simulink library "speedgoatlib_fpga_analog_io"  (R2024b)
settings: Solver=VariableStepAuto  StartTime=0.0  StopTime=10.0  RelTol=1e-3
undefined symbols (not defined in the file): IO336, sg_fpga_callBackInit_m_a1, sg_fpga_io324_analog_input_m, sg_fpga_io324_analog_output_m, sg_fpga_io324_analog_setup_m, sg_fpga_io325_analog_input_m, sg_fpga_io325_analog_output_m, sg_fpga_io325_analog_setup_m, sg_fpga_io334_analog_input_m, sg_fpga_io334_analog_output_m, sg_fpga_io334_analog_setup_m, sg_fpga_io336_analog_input_m, sg_fpga_io336_analog_output_m, sg_fpga_io336_analog_setup_m, sg_fpga_io337_analog_input_m, sg_fpga_io337_analog_output_m, sg_fpga_io337_analog_setup_m, sg_fpga_io3xx_120_analog_input_m, sg_fpga_io3xx_120_analog_output_m, sg_fpga_io3xx_120_analog_setup_m
(part 2 of 4)

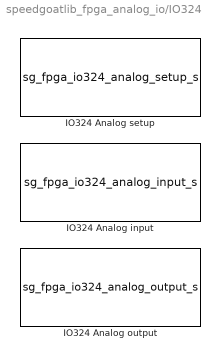
== system speedgoatlib_fpga_analog_io/IO324 ==
  IO324 Analog input : S-Function  InitFcn=sg_fpga_io324_analog_input_m.runInitFcn();  FunctionName=sg_fpga_io324_analog_input_s  Parameters=id, parSampleTime, parAiChannels, parAiVoltageRange, parAiTriggerMode, parAiReadPrevValue, parAiEnableFrame, parAiFrameSize  SFunctionDeploymentMode=off  EnableBusSupport=off  mask(ad_fpga_IO324){id=1, parSampleTime=-1, parPciSlot=-1, parAiChannels=[1 2], parAiTriggerMode=[2 2 2 2], parAiReadPrevValue=0, parAiEnableFrame=0, parAiVoltageRange=[3 3], parAdcCoupling=[1 1 1 1], parAdcContSampling=0, parAdcDmaEnable=0, parAdcActiveDmaDevices=[1 1 1 1], parAiFrameSize=100}
      mask prompts: id "Configurable I/O Module ID"; parSampleTime "Sample Time [s]"
      mask help: Speedgoat Driver Block<br>IO324-200k - IO324 Analog Input<br><br>&copy; 2007 - 2026, Speedgoat GmbH, <a href="matlab: web('www.speedgoat.com','-browser');">www.speedgoat.com</a>
      mask init:
      | sg_fpga_io324_analog_input_m.runMaskInit();
      mask Help: eval('sg.utils.help.show(''io_main/refentry_io324_analog_input_v1'');')
      mask TypeOptions id: 1 | 2 | 3 | 4 | 5 | 6 | 7 | 8 | 9 | 10
      mask Display: disp('Speedgoat\nIO324-200k\nAnalog input v1\nModule ID: 1');port_label('output',1,'1');port_label('output',2,'2');
  IO324 Analog output : S-Function  InitFcn=sg_fpga_io324_analog_output_m.runInitFcn();  FunctionName=sg_fpga_io324_analog_output_s  Parameters=id, parSampleTime, parAoChannels, parAoVoltageRange, parAoInitValues, parAoReset, parAoEnableFrame, parAoFrameSize  SFunctionDeploymentMode=off  EnableBusSupport=off  mask(da_fpga_IO324){id=1, parSampleTime=-1, parPciSlot=-1, parAoChannels=[1 2], parAoVoltageRange=[2 2], parDacOverRange=[0 0 0 0 0 0 0 0], parAoInitValues=[0 0], parAoReset=[1 1], parDacSyncOut=1, parAoEnableFrame=0, parDacActiveDmaDevices=[1 1 1 1], parDacDmaLatency=2, parAoFrameSize=1000}
      mask prompts: id "Configurable I/O Module ID"; parSampleTime "Sample Time [s]"
      mask help: Speedgoat Driver Block<br>IO324-200k - IO324 Analog Output<br><br>&copy; 2007 - 2026, Speedgoat GmbH, <a href="matlab: web('www.speedgoat.com','-browser');">www.speedgoat.com</a>
      mask init:
      | sg_fpga_io324_analog_output_m.runMaskInit();
      mask Help: eval('sg.utils.help.show(''io_main/refentry_io324_analog_output_v1'');')
      mask TypeOptions id: 1 | 2 | 3 | 4 | 5 | 6 | 7 | 8 | 9 | 10
      mask Display: disp('Speedgoat\nIO324-200k\nAnalog output v1\nModule ID: 1');port_label('input',1,'1');port_label('input',2,'2');
  IO324 Analog setup : S-Function  InitFcn=sg_fpga_io324_analog_setup_m.runInitFcn();  FunctionName=sg_fpga_io324_analog_setup_s  Parameters=id, p.AdcActiveChannels, p.AdcCoupling, p.AdcVoltageRange, p.AdcFilterWidthPow2, p.AdcOversamplRate, parAdcAutoCorrection, p.AdcTriggerMode, p.AdcClockDivider, p.AdcInternalTrigger, p.AdcExternalTrigger, p.AdcEnableFrame, p.AdcFrameSize, p.DacChannels, p.DacVoltageRange, p.DacInitValues, p.DacReset, parDacAutoCorrection, p.DacTriggerMode, p.DacClockDivider, p.DacInternalTrigger, p.DacExternalTrigger, p.DacEnableFrame, p.DacFifoThreshold, p.DacSourceSelection, p.EnableTriggerForCm,p.DacUsesTimer  SFunctionModules=sg_fpga_analog_dma sg_AnalogInputCm_IO324 sg_AnalogOutputCm  SFunctionDeploymentMode=off  EnableBusSupport=off  mask(analog_setup_fpga_IO324){id=1, parEnableCodeModule1=off, parEnableCodeModule2=off, parEnableCodeModule3=off, parEnableCodeModule4=off, parEnableCodeModule5=off, parEnableCodeModule6=off, parEnableCodeModule7=off, parEnableCodeModule8=off, parAdcEnableIndividualTrigger=off, parAdcTriggerMode1=Model Step, parAdcSampleRate1=100e3, parAdcDioTriggerChannel1=1, parAdcInternalTrigger1=<empty>, parAdcOversampling1=None, parAdcTriggerMode2=Model Step, parAdcSampleRate2=100e3, parAdcDioTriggerChannel2=1, parAdcInternalTrigger2=<empty>, parAdcOversampling2=None, parAdcTriggerMode3=Model Step, parAdcSampleRate3=100e3, parAdcDioTriggerChannel3=1, parAdcInternalTrigger3=<empty>, parAdcOversampling3=None, parAdcTriggerMode4=Model Step, parAdcSampleRate4=100e3, parAdcDioTriggerChannel4=1, parAdcInternalTrigger4=<empty>, parAdcOversampling4=None, parAdcReadPrevValueIndividualTrigger=on, parAdcEnableFrame=off, parAdcTriggerMode=I/O Module Clock, parAdcReadPrevValue=on, parAdcSampleRate=100e3, parAdcDioTriggerChannel=1, parAdcInternalTrigger=<empty>, parAdcOversampling=None, parAdcTriggerResolution=1e-08, parAdcSampleRateFrame=100e3, parAdcFrameSize=100, parAdcSampleTime=-1, parDacTriggerMode=Model Step, parDacInternalTrigger=<empty>, parDacDioTriggerChannel=0, parDacEnableFrame=on, dacUsesTimer=off, parDacFifoThreshold=100, parDacTriggerResolution=1e-08, parDacSampleRate=1e6, parDacFrameSize=1000, parDacSampleTime=-1, parAdcCoupling1=Single-Ended, parAdcChannel1=on, parAdcChannel2=on, parAdcChannel3=off, parAdcChannel4=off, parAdcChannel5=off, parAdcChannel6=off, parAdcChannel7=off, parAdcChannel8=off, parAdcRangeAll1=+-5.12 V, parVoltageRangePerChannelEn1=off, parAdcRange1=+-5.12 V, parAdcRange5=+-5.12 V, parAdcRange2=+-5.12 V, parAdcRange6=+-5.12 V, parAdcRange3=+-5.12 V, parAdcRange7=+-5.12 V, parAdcRange4=+-5.12 V, parAdcRange8=+-5.12 V, parAdcCoupling2=Single-Ended, parAdcChannel9=off, parAdcChannel10=off, parAdcChannel11=off, parAdcChannel12=off, parAdcChannel13=off, parAdcChannel14=off, parAdcChannel15=off, parAdcChannel16=off, parAdcRangeAll2=+-5.12 V, parVoltageRangePerChannelEn2=off, parAdcRange9=+-5.12 V, parAdcRange13=+-5.12 V, parAdcRange10=+-5.12 V, parAdcRange14=+-5.12 V, parAdcRange11=+-5.12 V, parAdcRange15=+-5.12 V, parAdcRange12=+-5.12 V, parAdcRange16=+-5.12 V, parAdcCoupling3=Single-Ended, parAdcChannel17=off, parAdcChannel18=off, parAdcChannel19=off, parAdcChannel20=off, parAdcChannel21=off, parAdcChannel22=off, parAdcChannel23=off, parAdcChannel24=off, parAdcRangeAll3=+-5.12 V, parVoltageRangePerChannelEn3=off, parAdcRange17=+-5.12 V, parAdcRange21=+-5.12 V, parAdcRange18=+-5.12 V, parAdcRange22=+-5.12 V, parAdcRange19=+-5.12 V, parAdcRange23=+-5.12 V, parAdcRange20=+-5.12 V, parAdcRange24=+-5.12 V, parAdcCoupling4=Single-Ended, parAdcChannel25=off, parAdcChannel26=off, parAdcChannel27=off, parAdcChannel28=off, parAdcChannel29=off, parAdcChannel30=off, parAdcChannel31=off, parAdcChannel32=off, parAdcRangeAll4=+-5.12 V, parVoltageRangePerChannelEn4=off, parAdcRange25=+-5.12 V, parAdcRange29=+-5.12 V, parAdcRange26=+-5.12 V, parAdcRange30=+-5.12 V, parAdcRange27=+-5.12 V, parAdcRange31=+-5.12 V, parAdcRange28=+-5.12 V, parAdcRange32=+-5.12 V, parAdcAutoCorrection=on, parDacChannel1=on, parDacChannel2=on, parDacChannel3=off, parDacChannel4=off, parDacChannel5=off, parDacChannel6=off, parDacChannel7=off, parDacChannel8=off, parDacRange1=+-5 V, parDacInitValue1=0, parDacReset1=on, parDacRange2=+-5 V, parDacInitValue2=0, parDacReset2=on, parDacRange3=+-5 V, parDacInitValue3=0, parDacReset3=on, parDacRange4=+-5 V, parDacInitValue4=0, parDacReset4=on, parDacRange5=+-5 V, parDacInitValue5=0, parDacReset5=on, parDacRange6=+-5 V, parDacInitValue6=0, parDacReset6=on, parDacRange7=+-5 V, parDacInitValue7=0, parDacReset7=on, parDacRange8=+-5 V, parDacInitValue8=0, parDacReset8=on, parDacAutoCorrection=on}
      mask prompts: id "Configurable I/O Module ID"; parAdcEnableIndividualTrigger "Enable Individual Trigger Settings"; parAdcTriggerMode1 "ADC Sample Trigger"; parAdcSampleRate1 "ADC Sample Rate [Hz]"; parAdcDioTriggerChannel1 "Digital I/O Channel"; parAdcInternalTrigger1 "Internal Signal"; parAdcOversampling1 "Oversampling Factor"; parAdcTriggerMode2 "ADC Sample Trigger"; parAdcSampleRate2 "ADC Sample Rate [Hz]"; parAdcDioTriggerChannel2 "Digital I/O Channel"; parAdcInternalTrigger2 "Internal Signal"; parAdcOversampling2 "Oversampling Factor"; parAdcTriggerMode3 "ADC Sample Trigger"; parAdcSampleRate3 "ADC Sample Rate [Hz]"; parAdcDioTriggerChannel3 "Digital I/O Channel"; parAdcInternalTrigger3 "Internal Signal"; parAdcOversampling3 "Oversampling Factor"; parAdcTriggerMode4 "ADC Sample Trigger"; parAdcSampleRate4 "ADC Sample Rate [Hz]"; parAdcDioTriggerChannel4 "Digital I/O Channel"; parAdcInternalTrigger4 "Internal Signal"; parAdcOversampling4 "Oversampling Factor"; parAdcReadPrevValueIndividualTrigger "Read Value From Previous Model Step"; parAdcEnableFrame "Enable DMA Interrupt"; parAdcTriggerMode "ADC Sample Trigger"; parAdcReadPrevValue "Read Value From Previous Model Step"; parAdcSampleRate "ADC Sample Rate [Hz]"; parAdcDioTriggerChannel "Digital I/O Channel"; parAdcInternalTrigger "Internal Signal"; parAdcOversampling "Oversampling Factor"; parAdcTriggerResolution "Trigger Resolution [s]"; parAdcSampleRateFrame "ADC Sample Rate [Hz]"; parAdcFrameSize "Frame Size (samples/channel)"; parAdcSampleTime "Input Block Sample Time [s]"; parDacTriggerMode "DAC Sample Trigger"; parDacInternalTrigger "Internal Signal"; parDacDioTriggerChannel "Digital I/O Channel"; parDacEnableFrame "Enable DMA Interrupt"; dacUsesTimer "Set Sampling Frequency"; parDacFifoThreshold "FIFO Threshold (samples/channel)"; parDacTriggerResolution "Trigger Resolution [s]"; parDacSampleRate "DAC Sample Rate [Hz]"; parDacFrameSize "Frame Size (samples/channel)"; parDacSampleTime "Output Block Sample Time [s]"; parAdcCoupling1 "Signal Mode"; parAdcChannel1 "Ch 01"; parAdcChannel2 "Ch 02"; parAdcChannel3 "Ch 03"; parAdcChannel4 "Ch 04"; parAdcChannel5 "Ch 05"; parAdcChannel6 "Ch 06"; parAdcChannel7 "Ch 07"; parAdcChannel8 "Ch 08"; parAdcRangeAll1 "Voltage Range"; parVoltageRangePerChannelEn1 "Set Voltage Range per Channel"; parAdcRange1 "Ch 01"; parAdcRange5 "Ch 05"; parAdcRange2 "Ch 02"; parAdcRange6 "Ch 06"; parAdcRange3 "Ch 03"; parAdcRange7 "Ch 07"; parAdcRange4 "Ch 04"; parAdcRange8 "Ch 08"; parAdcCoupling2 "Signal Mode"; parAdcChannel9 "Ch 09"; parAdcChannel10 "Ch 10"; parAdcChannel11 "Ch 11"; parAdcChannel12 "Ch 12"; parAdcChannel13 "Ch 13"; parAdcChannel14 "Ch 14"; parAdcChannel15 "Ch 15"; parAdcChannel16 "Ch 16"; parAdcRangeAll2 "Voltage Range"; parVoltageRangePerChannelEn2 "Set Voltage Range per Channel"; parAdcRange9 "Ch 09"; parAdcRange13 "Ch 13"; parAdcRange10 "Ch 10"; parAdcRange14 "Ch 14"; parAdcRange11 "Ch 11"; parAdcRange15 "Ch 15"; parAdcRange12 "Ch 12"; parAdcRange16 "Ch 16"; parAdcCoupling3 "Signal Mode"; parAdcChannel17 "Ch 17"; parAdcChannel18 "Ch 18"; parAdcChannel19 "Ch 19"; parAdcChannel20 "Ch 20"; parAdcChannel21 "Ch 21"; parAdcChannel22 "Ch 22"; parAdcChannel23 "Ch 23"; parAdcChannel24 "Ch 24"; parAdcRangeAll3 "Voltage Range"; parVoltageRangePerChannelEn3 "Set Voltage Range per Channel"; parAdcRange17 "Ch 17"; parAdcRange21 "Ch 21"; parAdcRange18 "Ch 18"; parAdcRange22 "Ch 22"; parAdcRange19 "Ch 19"; parAdcRange23 "Ch 23"; parAdcRange20 "Ch 20"; parAdcRange24 "Ch 24"; parAdcCoupling4 "Signal Mode"; parAdcChannel25 "Ch 25"; parAdcChannel26 "Ch 26"; parAdcChannel27 "Ch 27"; parAdcChannel28 "Ch 28"; parAdcChannel29 "Ch 29"; parAdcChannel30 "Ch 30"; parAdcChannel31 "Ch 31"; parAdcChannel32 "Ch 32"; parAdcRangeAll4 "Voltage Range"; parVoltageRangePerChannelEn4 "Set Voltage Range per Channel"; parAdcRange25 "Ch 25"; parAdcRange29 "Ch 29"; parAdcRange26 "Ch 26"; parAdcRange30 "Ch 30"; parAdcRange27 "Ch 27"; parAdcRange31 "Ch 31"; parAdcRange28 "Ch 28"; parAdcRange32 "Ch 32"; parAdcAutoCorrection "Automatic Data Correction (for Debugging)"; parDacChannel1 "Ch 1"; parDacChannel2 "Ch 2"; parDacChannel3 "Ch 3"; parDacChannel4 "Ch 4"; parDacChannel5 "Ch 5"; parDacChannel6 "Ch 6"; parDacChannel7 "Ch 7"; parDacChannel8 "Ch 8"; parDacRange1 "Output Range"; parDacInitValue1 "Initial Value [V]"; parDacReset1 "Reset to Initial Value"; parDacRange2 "Output Range"; parDacInitValue2 "Initial Value [V]"; parDacReset2 "Reset to Initial Value"; parDacRange3 "Output Range"; parDacInitValue3 "Initial Value [V]"; parDacReset3 "Reset to Initial Value"; parDacRange4 "Output Range"; parDacInitValue4 "Initial Value [V]"; parDacReset4 "Reset to Initial Value"; parDacRange5 "Output Range"; parDacInitValue5 "Initial Value [V]"; parDacReset5 "Reset to Initial Value"; parDacRange6 "Output Range"; parDacInitValue6 "Initial Value [V]"; parDacReset6 "Reset to Initial Value"; parDacRange7 "Output Range"; parDacInitValue7 "Initial Value [V]"; parDacReset7 "Reset to Initial Value"; parDacRange8 "Output Range"; parDacInitValue8 "Initial Value [V]"; parDacReset8 "Reset to Initial Value"; parDacAutoCorrection "Automatic Data Correction (for Debugging)"
      mask help: Speedgoat Driver Block<br>IO324-200k - IO324 Analog setup<br><br>&copy; 2007 - 2026, Speedgoat GmbH, <a href="matlab: web('www.speedgoat.com','-browser');">www.speedgoat.com</a>
      mask init:
      | p = sg_fpga_io324_analog_setup_m.runMaskInit();
      settings: OpenFcn=sg_fpga_io324_analog_setup_m.runOpenMaskCb();
      mask Help: eval('sg.utils.help.show(''io_main/refentry_io324_analog_setup_v1'');')
      mask TypeOptions id: 1 | 2 | 3 | 4 | 5 | 6 | 7 | 8 | 9 | 10
      mask Callback id: sg_fpga_io324_analog_setup_m.runModuleIdCb();
      mask Callback parEnableCodeModule1: sg_fpga_io324_analog_setup_m.runEnableCmCb(1);
      mask Callback parEnableCodeModule2: sg_fpga_io324_analog_setup_m.runEnableCmCb(2);
      mask Callback parEnableCodeModule3: sg_fpga_io324_analog_setup_m.runEnableCmCb(3);
      mask Callback parEnableCodeModule4: sg_fpga_io324_analog_setup_m.runEnableCmCb(4);
      mask Callback parEnableCodeModule5: sg_fpga_io324_analog_setup_m.runEnableCmCb(5);
      mask Callback parEnableCodeModule6: sg_fpga_io324_analog_setup_m.runEnableCmCb(6);
      mask Callback parEnableCodeModule7: sg_fpga_io324_analog_setup_m.runEnableCmCb(7);
      mask Callback parEnableCodeModule8: sg_fpga_io324_analog_setup_m.runEnableCmCb(8);
      mask Callback parAdcEnableIndividualTrigger: sg_fpga_io324_analog_setup_m.runAnalogInputCb();
      mask TypeOptions parAdcTriggerMode1: Model Step | I/O Module Clock | I/O Module Internal Signal | I/O Module Digital I/O
      mask Callback parAdcTriggerMode1: sg_fpga_io324_analog_setup_m.runAdcTriggerCb('suffix', '1');
      mask TypeOptions parAdcInternalTrigger1: <empty>
      mask TypeOptions parAdcOversampling1: None | 2 | 4 | 8 | 16 | 32 | 64
      mask TypeOptions parAdcTriggerMode2: Model Step | I/O Module Clock | I/O Module Internal Signal | I/O Module Digital I/O
      mask Callback parAdcTriggerMode2: sg_fpga_io324_analog_setup_m.runAdcTriggerCb('suffix', '2');
      mask TypeOptions parAdcInternalTrigger2: <empty>
      mask TypeOptions parAdcOversampling2: None | 2 | 4 | 8 | 16 | 32 | 64
      mask TypeOptions parAdcTriggerMode3: Model Step | I/O Module Clock | I/O Module Internal Signal | I/O Module Digital I/O
      mask Callback parAdcTriggerMode3: sg_fpga_io324_analog_setup_m.runAdcTriggerCb('suffix', '3');
      mask TypeOptions parAdcInternalTrigger3: <empty>
      mask TypeOptions parAdcOversampling3: None | 2 | 4 | 8 | 16 | 32 | 64
      mask TypeOptions parAdcTriggerMode4: Model Step | I/O Module Clock | I/O Module Internal Signal | I/O Module Digital I/O
      mask Callback parAdcTriggerMode4: sg_fpga_io324_analog_setup_m.runAdcTriggerCb('suffix', '4');
      mask TypeOptions parAdcInternalTrigger4: <empty>
      mask TypeOptions parAdcOversampling4: None | 2 | 4 | 8 | 16 | 32 | 64
      mask Callback parAdcEnableFrame: sg_fpga_io324_analog_setup_m.runEnableFrameCb();
      mask TypeOptions parAdcTriggerMode: Model Step | I/O Module Clock | I/O Module Internal Signal | I/O Module Digital I/O
      mask Callback parAdcTriggerMode: sg_fpga_io324_analog_setup_m.runAdcTriggerCb();
      mask TypeOptions parAdcInternalTrigger: <empty>
      mask TypeOptions parAdcOversampling: None | 2 | 4 | 8 | 16 | 32 | 64
      mask TypeOptions parDacTriggerMode: Model Step | I/O Module Clock | I/O Module Internal Signal | I/O Module Digital I/O
      mask Callback parDacTriggerMode: sg_fpga_io324_analog_setup_m.runDacTriggerCb();
      mask TypeOptions parDacInternalTrigger: <empty>
      mask Callback parDacEnableFrame: sg_fpga_io324_analog_setup_m.runDacTriggerCb();
      mask Callback dacUsesTimer: sg_fpga_io324_analog_setup_m.runDacTriggerCb();
      mask TypeOptions parAdcCoupling1: Single-Ended | Differential
      mask Callback parAdcCoupling1: sg_fpga_io324_analog_setup_m.runCouplingCb();
      mask Callback parAdcChannel1: sg_fpga_io324_analog_setup_m.runAnalogInputCb();
      mask Callback parAdcChannel2: sg_fpga_io324_analog_setup_m.runAnalogInputCb();
      mask Callback parAdcChannel3: sg_fpga_io324_analog_setup_m.runAnalogInputCb();
      mask Callback parAdcChannel4: sg_fpga_io324_analog_setup_m.runAnalogInputCb();
      mask Callback parAdcChannel5: sg_fpga_io324_analog_setup_m.runAnalogInputCb();
      mask Callback parAdcChannel6: sg_fpga_io324_analog_setup_m.runAnalogInputCb();
      mask Callback parAdcChannel7: sg_fpga_io324_analog_setup_m.runAnalogInputCb();
      mask Callback parAdcChannel8: sg_fpga_io324_analog_setup_m.runAnalogInputCb();
      mask TypeOptions parAdcRangeAll1: +-0.64 V | +-1.28 V | +-2.56 V | +-5.12 V | +-10.24 V | +-12.288 V (half resolution)
      mask Callback parVoltageRangePerChannelEn1: sg_fpga_io324_analog_setup_m.runAnalogInputCb();
      mask TypeOptions parAdcRange1: +-0.64 V | +-1.28 V | +-2.56 V | +-5.12 V | +-10.24 V | +-12.288 V (half resolution)
      mask TypeOptions parAdcRange5: +-0.64 V | +-1.28 V | +-2.56 V | +-5.12 V | +-10.24 V | +-12.288 V (half resolution)
      mask TypeOptions parAdcRange2: +-0.64 V | +-1.28 V | +-2.56 V | +-5.12 V | +-10.24 V | +-12.288 V (half resolution)
      mask TypeOptions parAdcRange6: +-0.64 V | +-1.28 V | +-2.56 V | +-5.12 V | +-10.24 V | +-12.288 V (half resolution)
      mask TypeOptions parAdcRange3: +-0.64 V | +-1.28 V | +-2.56 V | +-5.12 V | +-10.24 V | +-12.288 V (half resolution)
      mask TypeOptions parAdcRange7: +-0.64 V | +-1.28 V | +-2.56 V | +-5.12 V | +-10.24 V | +-12.288 V (half resolution)
      mask TypeOptions parAdcRange4: +-0.64 V | +-1.28 V | +-2.56 V | +-5.12 V | +-10.24 V | +-12.288 V (half resolution)
      mask TypeOptions parAdcRange8: +-0.64 V | +-1.28 V | +-2.56 V | +-5.12 V | +-10.24 V | +-12.288 V (half resolution)
      mask TypeOptions parAdcCoupling2: Single-Ended | Differential
      mask Callback parAdcCoupling2: sg_fpga_io324_analog_setup_m.runCouplingCb();
      mask Callback parAdcChannel9: sg_fpga_io324_analog_setup_m.runAnalogInputCb();
      mask Callback parAdcChannel10: sg_fpga_io324_analog_setup_m.runAnalogInputCb();
      mask Callback parAdcChannel11: sg_fpga_io324_analog_setup_m.runAnalogInputCb();
      mask Callback parAdcChannel12: sg_fpga_io324_analog_setup_m.runAnalogInputCb();
      mask Callback parAdcChannel13: sg_fpga_io324_analog_setup_m.runAnalogInputCb();
      mask Callback parAdcChannel14: sg_fpga_io324_analog_setup_m.runAnalogInputCb();
      mask Callback parAdcChannel15: sg_fpga_io324_analog_setup_m.runAnalogInputCb();
      mask Callback parAdcChannel16: sg_fpga_io324_analog_setup_m.runAnalogInputCb();
      mask TypeOptions parAdcRangeAll2: +-0.64 V | +-1.28 V | +-2.56 V | +-5.12 V | +-10.24 V | +-12.288 V (half resolution)
      mask Callback parVoltageRangePerChannelEn2: sg_fpga_io324_analog_setup_m.runAnalogInputCb();
      mask TypeOptions parAdcRange9: +-0.64 V | +-1.28 V | +-2.56 V | +-5.12 V | +-10.24 V | +-12.288 V (half resolution)
      mask TypeOptions parAdcRange13: +-0.64 V | +-1.28 V | +-2.56 V | +-5.12 V | +-10.24 V | +-12.288 V (half resolution)
      mask TypeOptions parAdcRange10: +-0.64 V | +-1.28 V | +-2.56 V | +-5.12 V | +-10.24 V | +-12.288 V (half resolution)
      mask TypeOptions parAdcRange14: +-0.64 V | +-1.28 V | +-2.56 V | +-5.12 V | +-10.24 V | +-12.288 V (half resolution)
      mask TypeOptions parAdcRange11: +-0.64 V | +-1.28 V | +-2.56 V | +-5.12 V | +-10.24 V | +-12.288 V (half resolution)
      mask TypeOptions parAdcRange15: +-0.64 V | +-1.28 V | +-2.56 V | +-5.12 V | +-10.24 V | +-12.288 V (half resolution)
      mask TypeOptions parAdcRange12: +-0.64 V | +-1.28 V | +-2.56 V | +-5.12 V | +-10.24 V | +-12.288 V (half resolution)
      mask TypeOptions parAdcRange16: +-0.64 V | +-1.28 V | +-2.56 V | +-5.12 V | +-10.24 V | +-12.288 V (half resolution)
      mask TypeOptions parAdcCoupling3: Single-Ended | Differential
      mask Callback parAdcCoupling3: sg_fpga_io324_analog_setup_m.runCouplingCb();
      mask Callback parAdcChannel17: sg_fpga_io324_analog_setup_m.runAnalogInputCb();
      mask Callback parAdcChannel18: sg_fpga_io324_analog_setup_m.runAnalogInputCb();
      mask Callback parAdcChannel19: sg_fpga_io324_analog_setup_m.runAnalogInputCb();
      mask Callback parAdcChannel20: sg_fpga_io324_analog_setup_m.runAnalogInputCb();
      mask Callback parAdcChannel21: sg_fpga_io324_analog_setup_m.runAnalogInputCb();
      mask Callback parAdcChannel22: sg_fpga_io324_analog_setup_m.runAnalogInputCb();
      mask Callback parAdcChannel23: sg_fpga_io324_analog_setup_m.runAnalogInputCb();
      mask Callback parAdcChannel24: sg_fpga_io324_analog_setup_m.runAnalogInputCb();
      mask TypeOptions parAdcRangeAll3: +-0.64 V | +-1.28 V | +-2.56 V | +-5.12 V | +-10.24 V | +-12.288 V (half resolution)
      mask Callback parVoltageRangePerChannelEn3: sg_fpga_io324_analog_setup_m.runAnalogInputCb();
      mask TypeOptions parAdcRange17: +-0.64 V | +-1.28 V | +-2.56 V | +-5.12 V | +-10.24 V | +-12.288 V (half resolution)
      mask TypeOptions parAdcRange21: +-0.64 V | +-1.28 V | +-2.56 V | +-5.12 V | +-10.24 V | +-12.288 V (half resolution)
      mask TypeOptions parAdcRange18: +-0.64 V | +-1.28 V | +-2.56 V | +-5.12 V | +-10.24 V | +-12.288 V (half resolution)
      mask TypeOptions parAdcRange22: +-0.64 V | +-1.28 V | +-2.56 V | +-5.12 V | +-10.24 V | +-12.288 V (half resolution)
      mask TypeOptions parAdcRange19: +-0.64 V | +-1.28 V | +-2.56 V | +-5.12 V | +-10.24 V | +-12.288 V (half resolution)
      mask TypeOptions parAdcRange23: +-0.64 V | +-1.28 V | +-2.56 V | +-5.12 V | +-10.24 V | +-12.288 V (half resolution)
      mask TypeOptions parAdcRange20: +-0.64 V | +-1.28 V | +-2.56 V | +-5.12 V | +-10.24 V | +-12.288 V (half resolution)
      mask TypeOptions parAdcRange24: +-0.64 V | +-1.28 V | +-2.56 V | +-5.12 V | +-10.24 V | +-12.288 V (half resolution)
      mask TypeOptions parAdcCoupling4: Single-Ended | Differential
      mask Callback parAdcCoupling4: sg_fpga_io324_analog_setup_m.runCouplingCb();
      mask Callback parAdcChannel25: sg_fpga_io324_analog_setup_m.runAnalogInputCb();
      mask Callback parAdcChannel26: sg_fpga_io324_analog_setup_m.runAnalogInputCb();
      mask Callback parAdcChannel27: sg_fpga_io324_analog_setup_m.runAnalogInputCb();
      mask Callback parAdcChannel28: sg_fpga_io324_analog_setup_m.runAnalogInputCb();
      mask Callback parAdcChannel29: sg_fpga_io324_analog_setup_m.runAnalogInputCb();
      mask Callback parAdcChannel30: sg_fpga_io324_analog_setup_m.runAnalogInputCb();
      mask Callback parAdcChannel31: sg_fpga_io324_analog_setup_m.runAnalogInputCb();
      mask Callback parAdcChannel32: sg_fpga_io324_analog_setup_m.runAnalogInputCb();
      mask TypeOptions parAdcRangeAll4: +-0.64 V | +-1.28 V | +-2.56 V | +-5.12 V | +-10.24 V | +-12.288 V (half resolution)
      mask Callback parVoltageRangePerChannelEn4: sg_fpga_io324_analog_setup_m.runAnalogInputCb();
      mask TypeOptions parAdcRange25: +-0.64 V | +-1.28 V | +-2.56 V | +-5.12 V | +-10.24 V | +-12.288 V (half resolution)
      mask TypeOptions parAdcRange29: +-0.64 V | +-1.28 V | +-2.56 V | +-5.12 V | +-10.24 V | +-12.288 V (half resolution)
      mask TypeOptions parAdcRange26: +-0.64 V | +-1.28 V | +-2.56 V | +-5.12 V | +-10.24 V | +-12.288 V (half resolution)
      mask TypeOptions parAdcRange30: +-0.64 V | +-1.28 V | +-2.56 V | +-5.12 V | +-10.24 V | +-12.288 V (half resolution)
      mask TypeOptions parAdcRange27: +-0.64 V | +-1.28 V | +-2.56 V | +-5.12 V | +-10.24 V | +-12.288 V (half resolution)
      mask TypeOptions parAdcRange31: +-0.64 V | +-1.28 V | +-2.56 V | +-5.12 V | +-10.24 V | +-12.288 V (half resolution)
      mask TypeOptions parAdcRange28: +-0.64 V | +-1.28 V | +-2.56 V | +-5.12 V | +-10.24 V | +-12.288 V (half resolution)
      mask TypeOptions parAdcRange32: +-0.64 V | +-1.28 V | +-2.56 V | +-5.12 V | +-10.24 V | +-12.288 V (half resolution)
      mask Callback parDacChannel1: sg_fpga_io324_analog_setup_m.runAnalogOutputCb();
      mask Callback parDacChannel2: sg_fpga_io324_analog_setup_m.runAnalogOutputCb();
      mask Callback parDacChannel3: sg_fpga_io324_analog_setup_m.runAnalogOutputCb();
      mask Callback parDacChannel4: sg_fpga_io324_analog_setup_m.runAnalogOutputCb();
      mask Callback parDacChannel5: sg_fpga_io324_analog_setup_m.runAnalogOutputCb();
      mask Callback parDacChannel6: sg_fpga_io324_analog_setup_m.runAnalogOutputCb();
      mask Callback parDacChannel7: sg_fpga_io324_analog_setup_m.runAnalogOutputCb();
      mask Callback parDacChannel8: sg_fpga_io324_analog_setup_m.runAnalogOutputCb();
      mask TypeOptions parDacRange1: +-2.5 V | +-5 V | +-10 V
      mask TypeOptions parDacRange2: +-2.5 V | +-5 V | +-10 V
      mask TypeOptions parDacRange3: +-2.5 V | +-5 V | +-10 V
      mask TypeOptions parDacRange4: +-2.5 V | +-5 V | +-10 V
      mask TypeOptions parDacRange5: +-2.5 V | +-5 V | +-10 V
      mask TypeOptions parDacRange6: +-2.5 V | +-5 V | +-10 V
      mask TypeOptions parDacRange7: +-2.5 V | +-5 V | +-10 V
      mask TypeOptions parDacRange8: +-2.5 V | +-5 V | +-10 V
      mask DialogControl tabMain Prompt: Main
      mask DialogControl boxModuleSettings Prompt: Module Settings
      mask DialogControl boxCodeModules Prompt: Code Module Functionality
      mask DialogControl boxAdcTrigger Prompt: Analog Input Trigger
      mask DialogControl boxAdcIndividualTrigger Prompt: Individual Trigger Settings (Sample Based)
      mask DialogControl boxAdcTrigger1 Prompt: Channel 01-08
      mask DialogControl boxAdcTrigger2 Prompt: Channel 09-16
      mask DialogControl boxAdcTrigger3 Prompt: Channel 17-24
      mask DialogControl boxAdcTrigger4 Prompt: Channel 25-32
      mask DialogControl boxAdcCommonTrigger Prompt: Common trigger settings
      mask DialogControl boxAdcFrameSettings Prompt: Frame-Based Settings
      mask DialogControl parAdcTriggerResolutionInfo Prompt: placeholder
      mask DialogControl parAdcSampleRateFrameInfo Prompt:
      | => 100 kHz
      | (10 us/sample)
      mask DialogControl parAdcFrameSizeInfo Prompt: => 100
      mask DialogControl parAdcSampleTimeInfo Prompt: => 1 ms
      mask DialogControl boxDacTrigger Prompt: Analog Output Trigger
      mask DialogControl boxDacFrameSettings Prompt: Frame-Based Settings
      mask DialogControl parDacFifoThresholdInfo Prompt: placeholder
      mask DialogControl parDacTriggerResolutionInfo Prompt: placeholder
      mask DialogControl parDacSampleRateInfo Prompt:
      | => 1 MHz
      | (1 us/sample)
      mask DialogControl parDacFrameSizeInfo Prompt: => 1000
      mask DialogControl parDacSampleTimeInfo Prompt: => 1 ms
      mask DialogControl tabAdc Prompt: Analog Inputs
      mask DialogControl boxAdc1 Prompt: Channel 01-08
      mask DialogControl parAdcAvailableChannels1 Prompt: Available Channels
      mask DialogControl boxAdc2 Prompt: Channel 09-16
      mask DialogControl parAdcAvailableChannels2 Prompt: Available Channels
      mask DialogControl boxAdc3 Prompt: Channel 17-24
      mask DialogControl parAdcAvailableChannels3 Prompt: Available Channels
      mask DialogControl boxAdc4 Prompt: Channel 25-32
      mask DialogControl parAdcAvailableChannels4 Prompt: Available Channels
      mask DialogControl tabDac Prompt: Analog Outputs
      mask DialogControl boxDacSetting Prompt: Channel Settings
      mask DialogControl boxDacChannels Prompt: Available Channels
      mask DialogControl boxDacChannel1 Prompt: Channel 1
      mask DialogControl boxDacChannel2 Prompt: Channel 2
      mask DialogControl boxDacChannel3 Prompt: Channel 3
      mask DialogControl boxDacChannel4 Prompt: Channel 4
      mask DialogControl boxDacChannel5 Prompt: Channel 5
      mask DialogControl boxDacChannel6 Prompt: Channel 6
      mask DialogControl boxDacChannel7 Prompt: Channel 7
      mask DialogControl boxDacChannel8 Prompt: Channel 8
      mask Display: disp('Speedgoat\nIO324-200k\nAnalog setup v1\nModule ID: 1');

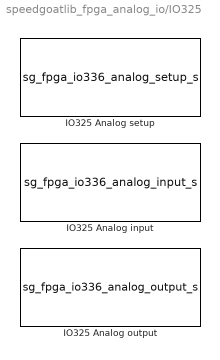
== system speedgoatlib_fpga_analog_io/IO325 ==
  IO325 Analog input : S-Function  InitFcn=sg_fpga_io325_analog_input_m.runInitFcn();  FunctionName=sg_fpga_io336_analog_input_s  Parameters=id, parSampleTime, parAiChannels, parAiChannelsStreamed, parAiVoltageRange, parAiTriggerMode, parAiReadPrevValue, parAiEnableFrame, parAiFrameSize  SFunctionDeploymentMode=off  EnableBusSupport=off  mask(ad_fpga_IO325){id=1, parSampleTime=-1, pciSlot=[-1,-1], parAiChannels=[1 2], parAiChannelsStreamed=[1 2], parAiTriggerMode=2, parAiReadPrevValue=0, parAiEnableFrame=0, parAiVoltageRange=[0 3 3 3], parAdcCoupling=[1 1 1 1], parAdcContSampling=0, parAdcDmaEnable=0, parAdcActiveDmaDevices=[1 1 1 1], parAiFrameSize=100}
      mask prompts: id "Configurable I/O Module ID"; parSampleTime "Sample Time [s]"
      mask help: Speedgoat Driver Block<br>IO325-160k - IO325 Analog Input<br><br>&copy; 2007 - 2026, Speedgoat GmbH, <a href="matlab: web('www.speedgoat.com','-browser');">www.speedgoat.com</a>
      mask init:
      | sg_fpga_io325_analog_input_m.runMaskInit();
      mask Help: eval('sg.utils.help.show(''io_main/refentry_io325_analog_input_v1'');')
      mask TypeOptions id: 1 | 2 | 3 | 4 | 5 | 6 | 7 | 8 | 9 | 10
      mask Display: disp('Speedgoat\nIO325-160k\nAnalog input v1\nModule ID: 1');port_label('output',1,'1');port_label('output',2,'2');
  IO325 Analog output : S-Function  InitFcn=sg_fpga_io325_analog_output_m.runInitFcn();  FunctionName=sg_fpga_io336_analog_output_s  Parameters=id, parSampleTime, parAoChannels, parAoVoltageRange, parAoInitValues, parAoReset, parAoEnableFrame, parAoFrameSize  SFunctionDeploymentMode=off  EnableBusSupport=off  mask(da_fpga_IO325){id=1, parSampleTime=-1, pciSlot=[-1,-1], board=IO336-325k, parAoChannels=[1 2], parAoVoltageRange=[1 1], parDacOverRange=[0 0 0 0 0 0 0 0], parAoInitValues=[0 0], parAoReset=[1 1], parDacSyncOut=1, parAoEnableFrame=0, parDacActiveDmaDevices=[1 1 1 1], parDacDmaLatency=2, parAoFrameSize=1000}
      mask prompts: id "Configurable I/O Module ID"; parSampleTime "Sample Time [s]"
      mask help: Speedgoat Driver Block<br>IO325-160k - IO325 Analog Output<br><br>&copy; 2007 - 2026, Speedgoat GmbH, <a href="matlab: web('www.speedgoat.com','-browser');">www.speedgoat.com</a>
      mask init:
      | sg_fpga_io325_analog_output_m.runMaskInit();
      mask Help: eval('sg.utils.help.show(''io_main/refentry_io325_analog_output_v1'');')
      mask TypeOptions id: 1 | 2 | 3 | 4 | 5 | 6 | 7 | 8 | 9 | 10
      mask Display: disp('Speedgoat\nIO325-160k\nAnalog output v1\nModule ID: 1');port_label('input',1,'1');port_label('input',2,'2');
  IO325 Analog setup : S-Function  InitFcn=sg_fpga_io325_analog_setup_m.runInitFcn();  FunctionName=sg_fpga_io336_analog_setup_s  Parameters=id, p.AdcActiveChannels, p.AdcVoltageRange, p.AdcFilterWidthPow2, p.AdcOversamplRate, parAdcAutoCorrection, p.AdcTriggerMode, p.AdcClockDivider, p.AdcInternalTrigger, p.AdcExternalTrigger, p.AdcEnableFrame, p.AdcFrameSize, p.DacChannels, p.DacVoltageRange, p.DacInitValues, p.DacReset, parDacAutoCorrection, p.DacTriggerMode, p.DacClockDivider, p.DacInternalTrigger, p.DacExternalTrigger, p.DacEnableFrame, p.DacFifoThreshold, p.DacSourceSelection, p.EnableTriggerForCm,p.DacUsesTimer  SFunctionModules=sg_fpga_analog_dma sg_AnalogInputCm_IO336 sg_AnalogOutputCm  SFunctionDeploymentMode=off  EnableBusSupport=off  mask(analog_setup_fpga_IO325){id=1, parEnableCodeModule1=off, parEnableCodeModule2=off, parEnableCodeModule3=off, parEnableCodeModule4=off, parEnableCodeModule5=off, parEnableCodeModule6=off, parEnableCodeModule7=off, parEnableCodeModule8=off, parAdcEnableIndividualTrigger=off, parAdcTriggerMode1=I/O Module Internal Signal, parAdcSampleRate1=100e3, parAdcDioTriggerChannel1=1, parAdcInternalTrigger1=<empty>, parAdcOversampling1=None, parAdcReadPrevValueIndividualTrigger=on, parAdcEnableFrame=off, parAdcTriggerMode=I/O Module Clock, parAdcReadPrevValue=on, parAdcSampleRate=100e3, parAdcDioTriggerChannel=1, parAdcInternalTrigger=<empty>, parAdcOversampling=None, parAdcTriggerResolution=1e-08, parAdcSampleRateFrame=100e3, parAdcFrameSize=100, parAdcSampleTime=-1, parDacTriggerMode=Model Step, parDacInternalTrigger=<empty>, parDacDioTriggerChannel=0, parDacEnableFrame=on, dacUsesTimer=off, parDacFifoThreshold=100, parDacTriggerResolution=1e-08, parDacSampleRate=1e6, parDacFrameSize=1000, parDacSampleTime=-1, parAdcChannel1=on, parAdcChannel2=on, parAdcChannel3=off, parAdcChannel4=off, parAdcChannel5=off, parAdcChannel6=off, parAdcChannel7=off, parAdcChannel8=off, parVoltageRangePerChannelEn1=off, parAdcRangeAll1=+/- 20V, parAdcRange1=+/- 20V, parAdcRange3=+/- 20V, parAdcRange2=+/- 20V, parAdcRange4=+/- 20V, parAdcAutoCorrection=on, parDacChannel1=on, parDacChannel2=on, parDacChannel3=off, parDacChannel4=off, parDacRange1=+-10 V, parDacInitValue1=0, parDacReset1=on, parDacRange2=+-10 V, parDacInitValue2=0, parDacReset2=on, parDacRange3=+-5 V, parDacInitValue3=0, parDacReset3=on, parDacRange4=+-5 V, parDacInitValue4=0, parDacReset4=on, parDacAutoCorrection=on}
      mask prompts: id "Configurable I/O Module ID"; parAdcEnableIndividualTrigger "Enable Individual Trigger Settings"; parAdcTriggerMode1 "ADC Sample Trigger"; parAdcSampleRate1 "ADC Sample Rate [Hz]"; parAdcDioTriggerChannel1 "Digital I/O Channel"; parAdcInternalTrigger1 "Internal Signal"; parAdcOversampling1 "Oversampling Factor"; parAdcReadPrevValueIndividualTrigger "Read Value From Previous Model Step"; parAdcEnableFrame "Enable DMA Interrupt"; parAdcTriggerMode "ADC Sample Trigger"; parAdcReadPrevValue "Read Value From Previous Model Step"; parAdcSampleRate "ADC Sample Rate [Hz]"; parAdcDioTriggerChannel "Digital I/O Channel"; parAdcInternalTrigger "Internal Signal"; parAdcOversampling "Oversampling Factor"; parAdcTriggerResolution "Trigger Resolution [s]"; parAdcSampleRateFrame "ADC Sample Rate [Hz]"; parAdcFrameSize "Frame Size (samples/channel)"; parAdcSampleTime "Input Block Sample Time [s]"; parDacTriggerMode "DAC Sample Trigger"; parDacInternalTrigger "Internal Signal"; parDacDioTriggerChannel "Digital I/O Channel"; parDacEnableFrame "Enable DMA Interrupt"; dacUsesTimer "Set Sampling Frequency"; parDacFifoThreshold "FIFO Threshold (samples/channel)"; parDacTriggerResolution "Trigger resolution [s]"; parDacSampleRate "DAC Sample Rate [Hz]"; parDacFrameSize "Frame Size (samples/channel)"; parDacSampleTime "Output Block Sample Time [s]"; parAdcChannel1 "Ch 01"; parAdcChannel2 "Ch 02"; parAdcChannel3 "Ch 03"; parAdcChannel4 "Ch 04"; parAdcChannel5 "Ch 05"; parAdcChannel6 "Ch 06"; parAdcChannel7 "Ch 07"; parAdcChannel8 "Ch 08"; parVoltageRangePerChannelEn1 "Set Voltage Range per Channel Pair"; parAdcRangeAll1 "Voltage Range"; parAdcRange1 "Ch 01 / 02"; parAdcRange3 "Ch 05 / 06"; parAdcRange2 "Ch 03 / 04"; parAdcRange4 "Ch 07 / 08"; parAdcAutoCorrection "Automatic Data Correction (for Debugging)"; parDacChannel1 "Ch 1"; parDacChannel2 "Ch 2"; parDacChannel3 "Ch 3"; parDacChannel4 "Ch 4"; parDacRange1 "Output Range"; parDacInitValue1 "Initial Value [V]"; parDacReset1 "Reset to Initial Value"; parDacRange2 "Output Range"; parDacInitValue2 "Initial Value [V]"; parDacReset2 "Reset to Initial Value"; parDacRange3 "Output Range"; parDacInitValue3 "Initial Value [V]"; parDacReset3 "Reset to Initial Value"; parDacRange4 "Output Range"; parDacInitValue4 "Initial Value [V]"; parDacReset4 "Reset to Initial Value"; parDacAutoCorrection "Automatic Data Correction (for Debugging)"
      mask help: Speedgoat Driver Block<br>IO325-160k - IO325 Analog setup<br><br>&copy; 2007 - 2026, Speedgoat GmbH, <a href="matlab: web('www.speedgoat.com','-browser');">www.speedgoat.com</a>
      mask init:
      | p = sg_fpga_io325_analog_setup_m.runMaskInit();
      settings: OpenFcn=sg_fpga_io325_analog_setup_m.runOpenMaskCb();
      mask Help: eval('sg.utils.help.show(''io_main/refentry_io325_analog_setup_v1'');')
      mask TypeOptions id: 1 | 2 | 3 | 4 | 5 | 6 | 7 | 8 | 9 | 10
      mask Callback id: sg_fpga_io325_analog_setup_m.runModuleIdCb();
      mask Callback parEnableCodeModule1: sg_fpga_io325_analog_setup_m.runEnableCmCb(1);
      mask Callback parEnableCodeModule2: sg_fpga_io325_analog_setup_m.runEnableCmCb(2);
      mask Callback parEnableCodeModule3: sg_fpga_io325_analog_setup_m.runEnableCmCb(3);
      mask Callback parEnableCodeModule4: sg_fpga_io325_analog_setup_m.runEnableCmCb(4);
      mask Callback parEnableCodeModule5: sg_fpga_io325_analog_setup_m.runEnableCmCb(5);
      mask Callback parEnableCodeModule6: sg_fpga_io325_analog_setup_m.runEnableCmCb(6);
      mask Callback parEnableCodeModule7: sg_fpga_io325_analog_setup_m.runEnableCmCb(7);
      mask Callback parEnableCodeModule8: sg_fpga_io325_analog_setup_m.runEnableCmCb(8);
      mask TypeOptions parAdcTriggerMode1: Model Step | I/O Module Clock | I/O Module Internal Signal | I/O Module Digital I/O
      mask Callback parAdcTriggerMode1: sg_fpga_io325_analog_setup_m.runAdcTriggerCb('suffix', '1')
      mask TypeOptions parAdcInternalTrigger1: <empty>
      mask TypeOptions parAdcOversampling1: None | 2 | 4 | 8 | 16 | 32 | 64
      mask Callback parAdcEnableFrame: sg_fpga_io325_analog_setup_m.runEnableFrameCb();
      mask TypeOptions parAdcTriggerMode: Model Step | I/O Module Clock | I/O Module Internal Signal | I/O Module Digital I/O
      mask Callback parAdcTriggerMode: sg_fpga_io325_analog_setup_m.runAdcTriggerCb();
      mask TypeOptions parAdcInternalTrigger: <empty>
      mask TypeOptions parAdcOversampling: None | 2 | 4 | 8 | 16 | 32 | 64
      mask TypeOptions parDacTriggerMode: Model Step | I/O Module Clock | I/O Module Internal Signal | I/O Module Digital I/O
      mask Callback parDacTriggerMode: sg_fpga_io325_analog_setup_m.runDacTriggerCb();
      mask TypeOptions parDacInternalTrigger: <empty>
      mask Callback parDacEnableFrame: sg_fpga_io325_analog_setup_m.runDacTriggerCb();
      mask Callback dacUsesTimer: sg_fpga_io325_analog_setup_m.runDacTriggerCb();
      mask Callback parAdcChannel1: sg_fpga_io325_analog_setup_m.runAnalogInputCb();
      mask Callback parAdcChannel2: sg_fpga_io325_analog_setup_m.runAnalogInputCb();
      mask Callback parAdcChannel3: sg_fpga_io325_analog_setup_m.runAnalogInputCb();
      mask Callback parAdcChannel4: sg_fpga_io325_analog_setup_m.runAnalogInputCb();
      mask Callback parAdcChannel5: sg_fpga_io325_analog_setup_m.runAnalogInputCb();
      mask Callback parAdcChannel6: sg_fpga_io325_analog_setup_m.runAnalogInputCb();
      mask Callback parAdcChannel7: sg_fpga_io325_analog_setup_m.runAnalogInputCb();
      mask Callback parAdcChannel8: sg_fpga_io325_analog_setup_m.runAnalogInputCb();
      mask Callback parVoltageRangePerChannelEn1: sg_fpga_io325_analog_setup_m.runAnalogInputCb();
      mask TypeOptions parAdcRangeAll1: +/- 20V | +/- 10V | +/- 5V
      mask TypeOptions parAdcRange1: +/- 20V | +/- 10V | +/- 5V
      mask TypeOptions parAdcRange3: +/- 20V | +/- 10V | +/- 5V
      mask TypeOptions parAdcRange2: +/- 20V | +/- 10V | +/- 5V
      mask TypeOptions parAdcRange4: +/- 20V | +/- 10V | +/- 5V
      mask Callback parDacChannel1: sg_fpga_io325_analog_setup_m.runAnalogOutputCb();
      mask Callback parDacChannel2: sg_fpga_io325_analog_setup_m.runAnalogOutputCb();
      mask Callback parDacChannel3: sg_fpga_io325_analog_setup_m.runAnalogOutputCb();
      mask Callback parDacChannel4: sg_fpga_io325_analog_setup_m.runAnalogOutputCb();
      mask TypeOptions parDacRange1: +-2.5 V | +-5 V | +-10 V
      mask TypeOptions parDacRange2: +-2.5 V | +-5 V | +-10 V
      mask TypeOptions parDacRange3: +-2.5 V | +-5 V | +-10 V
      mask TypeOptions parDacRange4: +-2.5 V | +-5 V | +-10 V
      mask DialogControl tabMain Prompt: Main
      mask DialogControl boxModuleSettings Prompt: Module Settings
      mask DialogControl boxCodeModules Prompt: Code Module Functionality
      mask DialogControl boxAdcTrigger Prompt: Analog Input Trigger
      mask DialogControl boxAdcIndividualTrigger Prompt: Individual Trigger Settings (Sample Based)
      mask DialogControl boxAdcTrigger1 Prompt: Channel 01-08
      mask DialogControl boxAdcCommonTrigger Prompt: Common Trigger Settings
      mask DialogControl boxAdcFrameSettings Prompt: Frame-Based Settings
      mask DialogControl parAdcTriggerResolutionInfo Prompt: placeholder
      mask DialogControl parAdcSampleRateFrameInfo Prompt:
      | => 100 kHz
      | (10 us/sample)
      mask DialogControl parAdcFrameSizeInfo Prompt: => 100
      mask DialogControl parAdcSampleTimeInfo Prompt: => 1 ms
      mask DialogControl boxDacTrigger Prompt: Analog Output Trigger
      mask DialogControl boxDacFrameSettings Prompt: Frame-Based Settings
      mask DialogControl parDacFifoThresholdInfo Prompt: placeholder
      mask DialogControl parDacTriggerResolutionInfo Prompt: placeholder
      mask DialogControl parDacSampleRateInfo Prompt:
      | => 1 MHz
      | (1 us/sample)
      mask DialogControl parDacFrameSizeInfo Prompt: => 1000
      mask DialogControl parDacSampleTimeInfo Prompt: => 1 ms
      mask DialogControl tabAdc Prompt: Analog Inputs
      mask DialogControl boxAdc1 Prompt: Channel 01-08
      mask DialogControl parAdcAvailableChannels1 Prompt: Available Channels
      mask DialogControl VoltageRangeBox1 Prompt: Individual voltage range
      mask DialogControl tabDac Prompt: Analog Outputs
      mask DialogControl boxDacSetting Prompt: Channel Settings
      mask DialogControl boxDacChannels Prompt: Available Channels
      mask DialogControl boxDacChannel1 Prompt: Channel 1
      mask DialogControl boxDacChannel2 Prompt: Channel 2
      mask DialogControl boxDacChannel3 Prompt: Channel 3
      mask DialogControl boxDacChannel4 Prompt: Channel 4
      mask Display: disp('Speedgoat\nIO325-160k\nAnalog setup v1\nModule ID: 1');

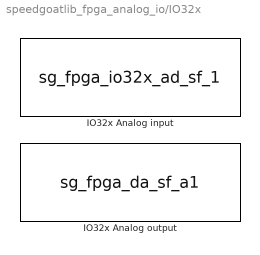
== system speedgoatlib_fpga_analog_io/IO32x ==
  IO32x Analog input : S-Function  InitFcn=sg_fpga_callBackInit_m_a1;  FunctionName=sg_fpga_io32x_ad_sf_1  Parameters="id, ts, ADC1_chan, ADC1_range, ADC1_diff, ADC1_Trigger, ADC1_Seq, ADC2_chan, ADC2_range, ADC2_diff, ADC2_Trigger, ADC2_Seq, ADC3_chan, ADC3_range, ADC3_diff, ADC3_Trigger, ADC3_Seq, ADC4_chan, ADC4_range,  ADC4_diff, ADC4_Trigger, ADC4_Seq"  SFunctionDeploymentMode=off  EnableBusSupport=off  mask(ad_IO32x_fpga_1){id=1, ts=0.001, ADC1_chan=[1:2], ADC1_range=+-10.24 V, ADC1_diff=Single-ended, ADC1_Trigger=Initiator, ADC1_Seq=on, ADC2_chan=[], ADC2_range=+-10.24 V, ADC2_diff=Differential, ADC2_Trigger=Initiator, ADC2_Seq=on, ADC3_chan=[], ADC3_range=+-10.24 V, ADC3_diff=Differential, ADC3_Trigger=Initiator, ADC3_Seq=on, ADC4_chan=[], ADC4_range=+-10.24 V, ADC4_diff=Differential, ADC4_Trigger=Initiator, ADC4_Seq=on}
      mask prompts: id "Configurable I/O Module ID"; ts "Sample time:"; ADC1_chan "Channel vector:"; ADC1_range "Range:"; ADC1_diff "Input coupling:"; ADC1_Trigger "Trigger mode:"; ADC1_Seq "Sequencer mode:"; ADC2_chan "Channel vector:"; ADC2_range "Range:"; ADC2_diff "Input coupling:"; ADC2_Trigger "Trigger mode:"; ADC2_Seq "Sequencer mode:"; ADC3_chan "Channel vector:"; ADC3_range "Range:"; ADC3_diff "Input coupling:"; ADC3_Trigger "Trigger mode:"; ADC3_Seq "Sequencer mode:"; ADC4_chan "Channel vector:"; ADC4_range "Range:"; ADC4_diff "Input coupling:"; ADC4_Trigger "Trigger mode:"; ADC4_Seq "Sequencer mode:"
      mask help: Speedgoat Driver Block<br>IO32x - Analog IO32x Input<br><br>&copy; 2007 - 2026, Speedgoat GmbH, <a href="matlab: web('www.speedgoat.com','-browser');">www.speedgoat.com</a>
      mask init:
      | sg_fpga_ad_io32x_m_1(id);
      mask Help: eval('sg.utils.help.show(''io_main/refentry_analog_io32x_input_v1'');')
      mask TypeOptions id: 1 | 2 | 3 | 4 | 5 | 6 | 7 | 8 | 9 | 10
      mask TypeOptions ADC1_range: +-24.576 V | +-20.48 V | +-10.24 V | +-5.12 V | +-2.56 V | +-1.28 V | +-0.64 V
      mask TypeOptions ADC1_diff: Single-ended | Differential
      mask TypeOptions ADC1_Trigger: Initiator | Target
      mask TypeOptions ADC2_range: +-24.576 V | +-20.48 V | +-10.24 V | +-5.12 V | +-2.56 V | +-1.28 V | +-0.64 V
      mask TypeOptions ADC2_diff: Single-ended | Differential
      mask TypeOptions ADC2_Trigger: Initiator | Target
      mask TypeOptions ADC3_range: +-24.576 V | +-20.48 V | +-10.24 V | +-5.12 V | +-2.56 V | +-1.28 V | +-0.64 V
      mask TypeOptions ADC3_diff: Single-ended | Differential
      mask TypeOptions ADC3_Trigger: Initiator | Target
      mask TypeOptions ADC4_range: +-24.576 V | +-20.48 V | +-10.24 V | +-5.12 V | +-2.56 V | +-1.28 V | +-0.64 V
      mask TypeOptions ADC4_diff: Single-ended | Differential
      mask TypeOptions ADC4_Trigger: Initiator | Target
      mask DialogControl ADC1_tab Prompt: ADC01
      mask DialogControl ADC1_text Prompt: ADC01  parameter settings:
      mask DialogControl ADC2_tab Prompt: ADC02
      mask DialogControl ADC2_text Prompt: ADC02  parameter settings:
      mask DialogControl ADC3_tab Prompt: ADC03
      mask DialogControl ADC3_text Prompt: ADC03  parameter settings:
      mask DialogControl ADC4_tab Prompt: ADC04
      mask DialogControl ADC4_text Prompt: ADC04  parameter settings:
      mask Display: disp('Speedgoat\nIO32x\nA/D read v1\nModule ID: 1');port_label('output', 1, 'ADC01 SE CH 1');port_label('output', 2, 'ADC01 SE CH 2');
  IO32x Analog output : S-Function  InitFcn=sg_fpga_callBackInit_m_a1;  FunctionName=sg_fpga_da_sf_a1  Parameters=id, chan, trigger, initVal, resetVal, ts  SFunctionDeploymentMode=off  EnableBusSupport=off  mask(da_IO32x_fpga_a1){id=1, chan=[1,2], trigger=Initiator, initVal=0, resetVal=0, ts=0.001, pciSlot=-1, board=Please select...}
      mask prompts: id "Configurable I/O Module ID"; chan "Channel vector:"; trigger "Trigger mode:"; initVal "Initial Values"; resetVal "Reset to Initial Values on model stop"; ts "Sample time:"; pciSlot "PCI slot (-1: autosearch):"
      mask help: Speedgoat Driver Block<br>IO32x - Analog IO32x Output<br><br>&copy; 2007 - 2026, Speedgoat GmbH, <a href="matlab: web('www.speedgoat.com','-browser');">www.speedgoat.com</a>
      mask init:
      | [boardType, initVal, resetVal] = sg_fpga_da_io32x_m_1(id);
      mask Help: eval('sg.utils.help.show(''io_main/refentry_analog_io32x_output_v1'');')
      mask TypeOptions id: 1 | 2 | 3 | 4 | 5 | 6 | 7 | 8 | 9 | 10
      mask TypeOptions trigger: Initiator | Target
      mask Display: disp('Speedgoat\nIO32x\nD/A write v1\nModule ID: 1');port_label('input', 1, '1');port_label('input', 2, '2');
